simulink model "question6_1_simulink"  (R2025b)
settings: Solver=ode45  StartTime=0.0  StopTime=2  RelTol=1e-3
settings Model: Creator=artes  LastModifiedBy=artes

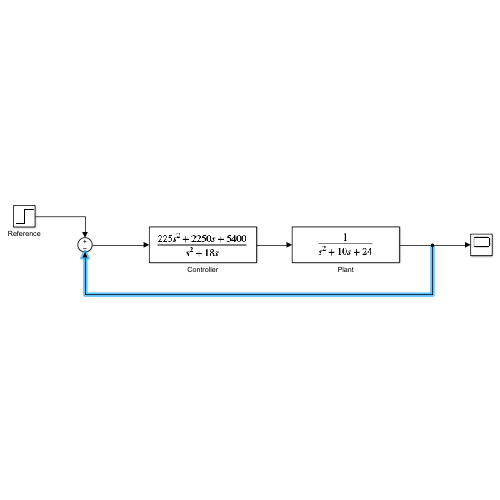
[thumbnail: Simulink's stored preview of the top-level diagram]
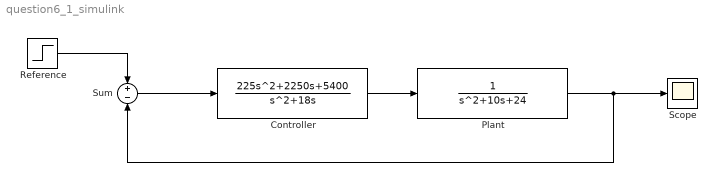
== system question6_1_simulink ==
  Controller : TransferFcn  Numerator=[225 2250 5400]  Denominator=[1 18 0]
  Plant : TransferFcn  Denominator=[1 10 24]
  Reference : Step  Time=0  SampleTime=0
  Scope : Scope
  Sum : Sum  Inputs=+-
  wires:
  Reference/1 -> Sum/1
  Sum/1 -> Controller/1
  Controller/1 -> Plant/1
  Plant/1 -> Scope/1, Sum/2
